simulink model "VehRT_211219"  (R2019b)
settings: Solver=ode5  StartTime=0.0  StopTime=Inf  FixedStep=Ts  RelTol=1e-3  EnableMultiTasking=on
InitFcn:
  | VehRT_Init_211219;
  | Ts=0.0005;
values from neighbouring files (symbols this model uses):
  damping_p = 0.113    [VehRT_Init_211219.m]
  Ff_ab_p = 0.41    [VehRT_Init_211219.m]
  Ff_c_p = 0.4    [VehRT_Init_211219.m]
  friction_enable = 1    [VehRT_Init_211219.m]
  sigma0_p = 200    [VehRT_Init_211219.m]
  sigma1_p = (200)^0.5    (= 14.1421356237)    [VehRT_Init_211219.m]
  td = 0.01    [VehRT_Init_211219.m]
  theta_sb_p = 0.03    [VehRT_Init_211219.m]
undefined symbols (not defined in the file or in its folder): C, canChannel, D, DiscIntNeverNeededParam, g, IO306, Kf, Kr, Lf, Lr, M, magnitude, sigma, trajectory_x11_, trajectory_x12_, trajectory_x13_, trajectory_x14_, trajectory_x15_, trajectory_x16_, trajectory_x17_, trajectory_x21_, trajectory_x22_, trajectory_x23_, trajectory_x24_, trajectory_x25_, trajectory_x26_, trajectory_x27_, trajectory_y11_, trajectory_y12_, trajectory_y13_, trajectory_y14_, trajectory_y15_, trajectory_y16_, trajectory_y17_, trajectory_y21_, trajectory_y22_, trajectory_y23_, trajectory_y24_, trajectory_y25_, trajectory_y26_, trajectory_y27_, zeta
libraries: canmsglib x31, speedgoatlib_IO612 x20, slrtlib x15, simulink x5, speedgoatlib_IO133 x3, xpcutilitieslib x2, canlib x2, xpcrtudplib x2, speedgoatlib_fpga x1, speedgoatlib_fpga_dio x1, autolibshared x1, speedgoatlib_fpga_quadrature x1
(part 3 of 4)

== system VehRT_211219/CEC Vehicle Dynamics 2021/CEC Vehicle Model 2021/ACC_controller ==
  note: V0.0.1 211028 xiataokai 简单PID-ACC速度控制器，0~1加速，-1~0制动
  des_spdKmph : Inport
  acc_mode : Inport  Port=2
  thr_m : Inport  Port=3
  brk_m : Inport  Port=4
  real_spdKmph : Inport  Port=5
  ACC_PID : simulink/Continuous/PID Controller  Controller=PID  Form=Parallel  TimeDomain=Discrete-time  SampleTime=-1  IntegratorMethod=Forward Euler  FilterMethod=Forward Euler  ControllerParametersSource=internal  P=0.11  I=0  D=0.04  UseFilter=on  N=100  TunerSelectOption=Transfer Function Based (PID Tuner App)  InitialConditionSource=internal  InitialConditionForIntegrator=0  InitialConditionForFilter=0  DifferentiatorICPrevScaledInput=0  ExternalReset=none  TrackingMode=off  Kt=1  LimitOutput=on  UpperSaturationLimit=1  LowerSaturationLimit=-2  LinearizeAsGain=on  AntiWindupMode=none  Kb=1  POutMin=[]  POutMax=[]  IOutMin=[]  IOutMax=[]  DOutMin=[]  DOutMax=[]  NOutMin=[]  NOutMax=[]  SumOutMin=[]  SumOutMax=[]  SaturationOutMin=[]  SaturationOutMax=[]  PParamMin=[]  PParamMax=[]  IParamMin=[]  IParamMax=[]  DParamMin=[]  DParamMax=[]  NParamMin=[]  NParamMax=[]  KbParamMin=[]  KbParamMax=[]  KtParamMin=[]  KtParamMax=[]  KbOutMin=[]  KbOutMax=[]  KtOutMin=[]  KtOutMax=[]  IntegratorOutMin=[]  IntegratorOutMax=[]  FilterOutMin=[]  FilterOutMax=[]  SumI1OutMin=[]  SumI1OutMax=[]  SumI2OutMin=[]  SumI2OutMax=[]  SumI3OutMin=[]  SumI3OutMax=[]  SumI4OutMin=[]  SumI4OutMax=[]  SumDOutMin=[]  SumDOutMax=[]  DifferentiatorOutMin=[]  DifferentiatorOutMax=[]  FilterDiffOutCoefMin=[]  FilterDiffOutCoefMax=[]  ReciprocalOutMin=[]  ReciprocalOutMax=[]  SumDenOutMin=[]  SumDenOutMax=[]  SumNumOutMin=[]  SumNumOutMax=[]  DivideOutMin=[]  DivideOutMax=[]  IntegratorContinuousStateAttributes=''  IntegratorStateMustResolveToSignalObject=off  IntegratorRTWStateStorageClass=Auto  FilterContinuousStateAttributes=''  FilterStateMustResolveToSignalObject=off  FilterRTWStateStorageClass=Auto  ParallelPVariant=InternalParameters  IdealPVariant=Disabled  IVariant=InternalParameters  DVariant=InternalParameters  IntegratorVariant=Discrete  SatVariant=Enabled  AWVariant=Passthrough  PCopyVariant=Disabled  TRVariant=Disabled  FdbkBlocksVariant=Forward  IdealPFdbkVariant=Disabled  SatFdbkVariant=Disabled  DerivativeFilterVariant=ForwardEulerFilter  NVariant=InternalParameters  NCopyVariant=Disabled  FilterICVariant=InternalICsFilter  IntegratorICVariant=InternalICs  ExternalResetVariant=Disabled  TRSumVariant=Passthrough  SumFdbkVariant=Disabled  SumVariant=Sum_PID
  Add : Sum  Inputs=+-
  Constant : Constant  Value=0
  Constant1 : Constant  Value=0
  Constant2 : Constant  Value=0
  Gain_brk : Gain  Gain=-1
  Gain_thr : Gain
  LPF : TransferFcn  Denominator=[1/2/pi/1.5 1]
  LT_brk : Lookup_n-D  NumberOfTableDimensions=1  BreakpointsForDimension1=[0, 0.3, 1]  Table=[0, 0.1, 1]  InternalRulePriority=Speed  RndMeth=Simplest  InputSameDT=on
  Switch : Switch  Criteria=u2 > Threshold
  Switch1 : Switch  Criteria=u2 > Threshold
  Switch2 : Switch  Criteria=u2 > Threshold
  Switch_brk : Switch  Criteria=u2 > Threshold
  Switch_thr : Switch  Criteria=u2 > Threshold
  max1_1 : Saturate  UpperLimit=1  LowerLimit=0
  max1_2 : Saturate  UpperLimit=1  LowerLimit=0
  open_loop_comp : Gain  Gain=1.02
  thr : Outport
  brk : Outport  Port=2
  wires:
  des_spdKmph/1 -> open_loop_comp/1
  real_spdKmph/1 -> Add/2
  Add/1 -> Switch/1
  ACC_PID/1 -> LPF/1
  Constant/1 -> Switch_brk/1
  Constant1/1 -> Switch_thr/3
  Switch_brk/1 -> Gain_brk/1
  Gain_brk/1 -> LT_brk/1
  Switch_thr/1 -> Gain_thr/1
  max1_1/1 -> Switch1/1
  Gain_thr/1 -> max1_2/1
  max1_2/1 -> Switch2/1
  LT_brk/1 -> max1_1/1
  LPF/1 -> Switch_thr/1, Switch_thr/2, Switch_brk/3, Switch_brk/2
  open_loop_comp/1 -> Add/1
  Switch/1 -> ACC_PID/1
  Constant2/1 -> Switch/3
  acc_mode/1 -> Switch2/2, Switch1/2, Switch/2
  thr_m/1 -> Switch2/3
  Switch2/1 -> thr/1
  Switch1/1 -> brk/1
  brk_m/1 -> Switch1/3

== system VehRT_211219/CEC Vehicle Dynamics 2021/CEC Vehicle Model 2021/Allocating_T_b ==
  T_brk : Inport
  Selector : Selector  InputPortWidth=4  IndexOptions=Index vector (dialog)  Indices=[1]  OutputSizes=1
  Selector1 : Selector  InputPortWidth=4  IndexOptions=Index vector (dialog)  Indices=[2]  OutputSizes=1
  Selector2 : Selector  InputPortWidth=4  IndexOptions=Index vector (dialog)  Indices=[3]  OutputSizes=1
  Selector3 : Selector  InputPortWidth=4  IndexOptions=Index vector (dialog)  Indices=[4]  OutputSizes=1
  Vector Concatenate : Concatenate  NumInputs=4
  T_b : Outport
  wires:
  Vector Concatenate/1 -> T_b/1
  Selector2/1 -> Vector Concatenate/3
  Selector3/1 -> Vector Concatenate/4
  Selector/1 -> Vector Concatenate/1
  Selector1/1 -> Vector Concatenate/2
  T_brk/1 -> Selector3/1, Selector2/1, Selector/1, Selector1/1

== system VehRT_211219/CEC Vehicle Dynamics 2021/CEC Vehicle Model 2021/Allocating_T_d ==
  T_drv : Inport
  Constant : Constant  Value=0
  Constant1 : Constant  Value=0
  Selector : Selector  InputPortWidth=2  IndexOptions=Index vector (dialog)  Indices=[1]  OutputSizes=1
  Selector1 : Selector  InputPortWidth=2  IndexOptions=Index vector (dialog)  Indices=[2]  OutputSizes=1
  Vector Concatenate : Concatenate  NumInputs=4
  T_d : Outport
  wires:
  Vector Concatenate/1 -> T_d/1
  T_drv/1 -> Selector1/1, Selector/1
  Selector/1 -> Vector Concatenate/1
  Selector1/1 -> Vector Concatenate/2
  Constant/1 -> Vector Concatenate/3
  Constant1/1 -> Vector Concatenate/4

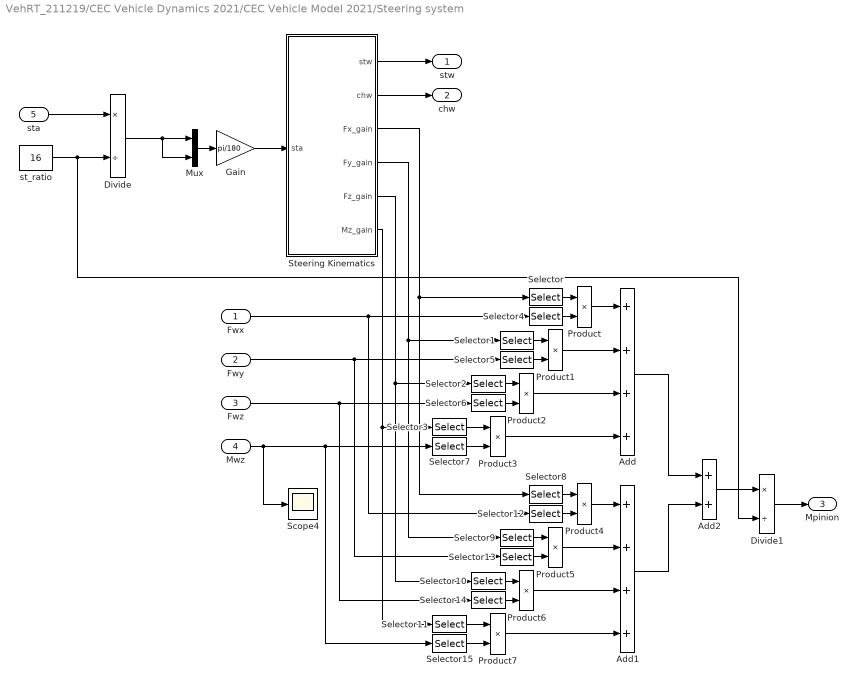
== system VehRT_211219/CEC Vehicle Dynamics 2021/CEC Vehicle Model 2021/Steering system ==
  Fwx : Inport
  Fwy : Inport  Port=2
  Fwz : Inport  Port=3
  Mwz : Inport  Port=4
  sta : Inport  Port=5
  Add : Sum  Inputs=++++
  Add1 : Sum  Inputs=++++
  Add2 : Sum
  Divide : Product  Inputs=*/
  Divide1 : Product  Inputs=*/
  Gain : Gain  Gain=pi/180
  Mux : Mux  Inputs=2
  Product{,1..7} (8 alike) : Product
  Scope4 : Scope
  Selector{,1..3} (4 alike) : Selector  InputPortWidth=2  IndexOptions=Index vector (dialog)  Indices=[1]  OutputSizes=1
  Selector{8..11} (4 alike) : Selector  InputPortWidth=2  IndexOptions=Index vector (dialog)  Indices=[2]  OutputSizes=1
  Selector{12..15} (4 alike) : Selector  InputPortWidth=4  IndexOptions=Index vector (dialog)  Indices=[2]  OutputSizes=1
  Selector{4..7} (4 alike) : Selector  InputPortWidth=4  IndexOptions=Index vector (dialog)  Indices=[1]  OutputSizes=1
  Steering Kinematics : MATLAB Function
  st_ratio : Constant  Value=16
  stw : Outport
  chw : Outport  Port=2
  Mpinion : Outport  Port=3
  wires:
  Gain/1 -> Steering Kinematics/1(sta)
  Mux/1 -> Gain/1
  Divide/1 -> Mux/2, Mux/1
  sta/1 -> Divide/1
  st_ratio/1 -> Divide1/2, Divide/2
  Steering Kinematics/1(stw) -> stw/1
  Steering Kinematics/2(chw) -> chw/1
  Fwx/1 -> Selector12/1, Selector4/1
  Steering Kinematics/3(Fx_gain) -> Selector8/1, Selector/1
  Steering Kinematics/5(Fz_gain) -> Selector10/1, Selector2/1
  Fwz/1 -> Selector14/1, Selector6/1
  Steering Kinematics/6(Mz_gain) -> Selector11/1, Selector3/1
  Mwz/1 -> Scope4/1, Selector15/1, Selector7/1
  Product3/1 -> Add/4
  Product/1 -> Add/1
  Product1/1 -> Add/2
  Product2/1 -> Add/3
  Add/1 -> Add2/1
  Selector/1 -> Product/1
  Selector1/1 -> Product1/1
  Selector2/1 -> Product2/1
  Selector3/1 -> Product3/1
  Selector4/1 -> Product/2
  Selector5/1 -> Product1/2
  Selector6/1 -> Product2/2
  Selector7/1 -> Product3/2
  Add1/1 -> Add2/2
  Selector11/1 -> Product7/1
  Selector12/1 -> Product4/2
  Product6/1 -> Add1/3
  Selector13/1 -> Product5/2
  Selector15/1 -> Product7/2
  Selector9/1 -> Product5/1
  Selector8/1 -> Product4/1
  Selector14/1 -> Product6/2
  Selector10/1 -> Product6/1
  Product7/1 -> Add1/4
  Product4/1 -> Add1/1
  Product5/1 -> Add1/2
  Add2/1 -> Divide1/1
  Steering Kinematics/4(Fy_gain) -> Selector9/1, Selector1/1
  Fwy/1 -> Selector13/1, Selector5/1
  Divide1/1 -> Mpinion/1

== system VehRT_211219/CEC Vehicle Dynamics 2021/CEC Vehicle Model 2021/Vehicle_initializer ==
  spd0Kmph : Inport
  MATLAB Function : MATLAB Function  TreatAsAtomicUnit=on
  pwrXInit : Outport
  gearInit : Outport  Port=2
  tirInit : Outport  Port=3
  vehInit : Outport  Port=4
  wires:
  spd0Kmph/1 -> MATLAB Function/1(V)
  MATLAB Function/1(gearInit) -> gearInit/1
  MATLAB Function/3(pwrXInit) -> pwrXInit/1
  MATLAB Function/4(tirXInit) -> tirInit/1
  MATLAB Function/2(vehXInit) -> vehInit/1

== system VehRT_211219/CEC Vehicle Dynamics 2021/CEC Vehicle Model 2021/awCal ==
  In1 : Inport
  Selector_aw : Selector  InputPortWidth=8  IndexOptions=Index vector (dialog)  Indices=[5:8]  OutputSizes=1
  atan_and_r2d : MATLAB Function  TreatAsAtomicUnit=on
  y : Outport
  wires:
  In1/1 -> Selector_aw/1
  Selector_aw/1 -> atan_and_r2d/1(u)
  atan_and_r2d/1(y) -> y/1

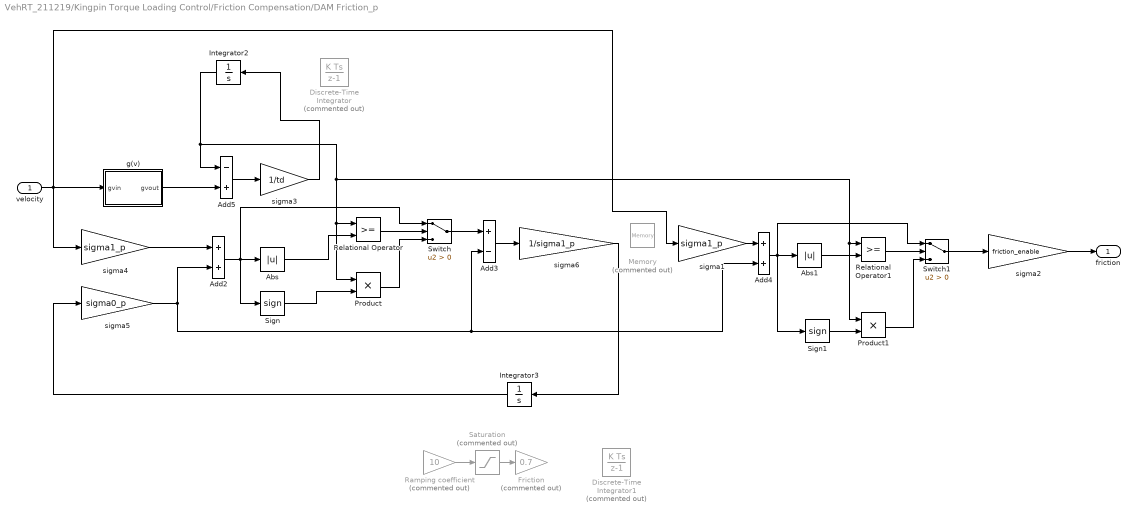
== system VehRT_211219/Kingpin Torque Loading Control/Friction Compensation/DAM Friction_p ==
  velocity : Inport
  Abs : Abs
  Abs1 : Abs
  Add2 : Sum
  Add3 : Sum  Inputs=+-
  Add4 : Sum
  Add5 : Sum  Inputs=-+
  Discrete-Time Integrator : DiscreteIntegrator  Commented=on  SampleTime=-1  ICPrevOutput=DiscIntNeverNeededParam  ICPrevScaledInput=DiscIntNeverNeededParam
  Discrete-Time Integrator1 : DiscreteIntegrator  Commented=on  SampleTime=-1  LimitOutput=on  UpperSaturationLimit=Ff_ab_p/sigma0_p  LowerSaturationLimit=-Ff_ab_p/sigma0_p  ICPrevOutput=DiscIntNeverNeededParam  ICPrevScaledInput=DiscIntNeverNeededParam
  Friction : Gain  Commented=on  Gain=0.7
  Integrator2 : Integrator
  Integrator3 : Integrator  LimitOutput=on  UpperSaturationLimit=Ff_ab_p/sigma0_p  LowerSaturationLimit=-Ff_ab_p/sigma0_p
  Memory : Memory  Commented=on
  Product : Product  RndMeth=Zero
  Product1 : Product  RndMeth=Zero
  Ramping coefficient : Gain  Commented=on  Gain=10
  Relational Operator : RelationalOperator  OutDataTypeStr=boolean  RndMeth=Nearest
  Relational Operator1 : RelationalOperator  OutDataTypeStr=boolean  RndMeth=Nearest
  Saturation : Saturate  Commented=on  UpperLimit=1  LowerLimit=-1
  Sign : Signum
  Sign1 : Signum
  Switch : Switch  Criteria=u2 > Threshold
  Switch1 : Switch  Criteria=u2 > Threshold
  g(v) : Subsystem
  sigma1 : Gain  Gain=sigma1_p
  sigma2 : Gain  Gain=friction_enable
  sigma3 : Gain  Gain=1/td
  sigma4 : Gain  Gain=sigma1_p
  sigma5 : Gain  Gain=sigma0_p
  sigma6 : Gain  Gain=1/sigma1_p
  friction : Outport  VectorParamsAs1DForOutWhenUnconnected=off
  wires:
  Relational Operator1/1 -> Switch1/2
  Abs1/1 -> Relational Operator1/2
  sigma1/1 -> Add4/1
  Integrator3/1 -> sigma5/1
  Add3/1 -> sigma6/1
  Switch/1 -> Add3/1
  Product/1 -> Switch/3
  Sign/1 -> Product/2
  Relational Operator/1 -> Switch/2
  Abs/1 -> Relational Operator/2
  Add2/1 -> Sign/1, Switch/1, Abs/1
  sigma6/1 -> Integrator3/1
  sigma5/1 -> Add2/2, Add3/2, Add4/2
  sigma4/1 -> Add2/1
  Add5/1 -> sigma3/1
  g(v)/1(gvout) -> Add5/2
  Switch1/1 -> sigma2/1
  sigma2/1 -> friction/1
  sigma3/1 -> Integrator2/1
  velocity/1 -> sigma1/1, sigma4/1, g(v)/1(gvin)
  Product1/1 -> Switch1/3
  Sign1/1 -> Product1/2
  Add4/1 -> Sign1/1, Switch1/1, Abs1/1
  Integrator2/1 -> Product1/1, Relational Operator1/1, Product/1, Relational Operator/1, Add5/1
  Saturation/1 -> Friction/1
  Ramping coefficient/1 -> Saturation/1

== system VehRT_211219/Kingpin Torque Loading Control/Old baks/Aligning Torque Calculator ==
  Beta : Inport
  r : Inport  Port=2
  Fzf : Inport  Port=3
  speed : Inport  Port=4
  Delta : Inport  Port=5
  Add3 : Sum  Inputs=++-
  Add4 : Sum
  Divide1 : Product  Inputs=*/
  Divide2 : Product  Inputs=**
  Gain : Gain  Gain=2
  Gain1 : Gain  Gain=Lf
  Gain2 : Gain  Gain=2*zeta*Kf
  Gain5 : Gain  Gain=0.5*D*sin(2*sigma)
  Trigonometric Function : Trigonometry
  Tire Aligning Torque : Outport  VectorParamsAs1DForOutWhenUnconnected=off
  wires:
  r/1 -> Gain1/1
  Gain1/1 -> Divide1/1
  speed/1 -> Divide1/2
  Delta/1 -> Trigonometric Function/1, Add3/3  "Delta"
  Beta/1 -> Add3/2
  Divide1/1 -> Add3/1
  Add3/1 -> Gain2/1
  Trigonometric Function/1 -> Divide2/1
  Divide2/1 -> Gain5/1
  Gain2/1 -> Add4/1
  Gain5/1 -> Add4/2
  Add4/1 -> Tire Aligning Torque/1
  Gain/1 -> Divide2/2
  Fzf/1 -> Gain/1

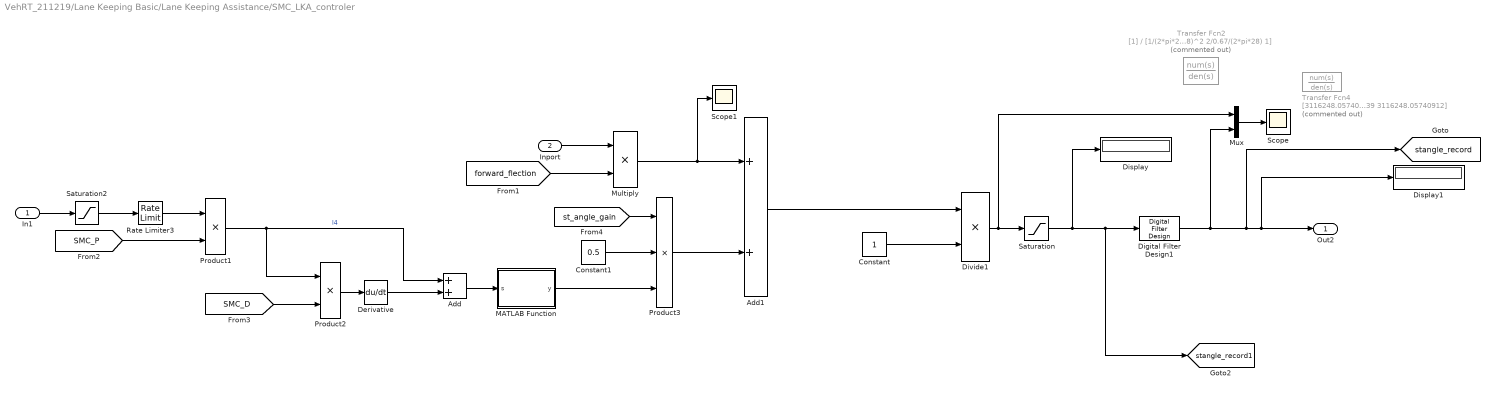
== system VehRT_211219/Lane Keeping Basic/Lane Keeping Assistance/SMC_LKA_controler ==
  In1 : Inport
  Inport : Inport  Port=2
  Add : Sum
  Add1 : Sum
  Constant : Constant
  Constant1 : Constant  Value=0.5
  Derivative : Derivative
  Digital Filter Design1 : dsparch4/Digital Filter Design  mwdsp_browser_bugfix_var=off
  Display : Display
  Display1 : Display
  Divide1 : Product  Inputs=**
  MATLAB Function : MATLAB Function  TreatAsAtomicUnit=on
  Multiply : Product
  Mux : Mux  Inputs=2
  Product1 : Product
  Product2 : Product
  Product3 : Product  Inputs=3
  Rate Limiter3 : RateLimiter  RisingSlewLimit=25  FallingSlewLimit=-25  SampleTimeMode=inherited
  Saturation : Saturate  UpperLimit=60  LowerLimit=-60
  Saturation2 : Saturate  UpperLimit=4  LowerLimit=-4
  Scope : Scope
  Scope1 : Scope
  Transfer Fcn2 : TransferFcn  Commented=on  Denominator=[1/(2*pi*28)^2 2/0.67/(2*pi*28) 1]
  Transfer Fcn4 : TransferFcn  Commented=on  Numerator=[3116248.05740912]  Denominator=[1 292.128549685798 42669.5447707639 3116248.05740912]
  Out2 : Outport  VectorParamsAs1DForOutWhenUnconnected=off
  tag scope: stangle_record1=global, stangle_record=global
  wires:
  Product3/1 -> Add1/2
  Add/1 -> MATLAB Function/1(s)
  Derivative/1 -> Add/2
  Product1/1 -> Add/1, Product2/1  "l4"
  Product2/1 -> Derivative/1
  [SMC_D] -> Product2/2
  Constant1/1 -> Product3/2
  [st_angle_gain] -> Product3/1
  MATLAB Function/1(y) -> Product3/3
  Add1/1 -> Divide1/1
  Divide1/1 -> Saturation/1, Mux/1
  Mux/1 -> Scope/1
  Constant/1 -> Divide1/2
  Multiply/1 -> Scope1/1, Add1/1
  Inport/1 -> Multiply/1
  [SMC_P] -> Product1/2
  Saturation2/1 -> Rate Limiter3/1
  In1/1 -> Saturation2/1
  [forward_flection] -> Multiply/2
  Rate Limiter3/1 -> Product1/1
  Digital Filter Design1/1 -> [stangle_record], Display1/1, Out2/1, Mux/2
  Saturation/1 -> Digital Filter Design1/1, [stangle_record1], Display/1

== system VehRT_211219/Lane Keeping Basic/Lane Keeping Assistance/signal processing ==
  Demux : Demux  Outputs=2
  Display : Display
  Gain : Gain
  Mux : Mux  Inputs=2
  Mux1 : Mux  Inputs=2
  Relational Operator : RelationalOperator  Operator=>  OutDataTypeStr=boolean  RndMeth=Simplest
  Saturation : Saturate  UpperLimit=4  LowerLimit=-4
  Switch : Switch  Criteria=u2 > Threshold  Threshold=0.5
  loading scope : slrtlib/Displays and Logging/Scope   scopeno=2  scopetype=Target  autostart=on  viewmode=Graphical rolling  formatstr='%15.6f'  grid=on  ylimits=[-5,5]  nosamples=1000  noprepostsamples=0  interleave=1  triggermode=FreeRun  triggersignal=1  trigsignalfromport=off  triggerlevel=0.0  triggerslope=Either  triggerscope=1  triggersample=0  filename=data.dat  mode=Lazy  writesize=512  autorestart=off  dynamicfilemode=off  maxwritefilesize=512*1024^2
  path_following : MATLAB Function  TreatAsAtomicUnit=on
  prepoint_y : Subsystem
  offset_at_prviewtime1 : Outport  VectorParamsAs1DForOutWhenUnconnected=off
  qulv_at_prviewtime2 : Outport  Port=2  VectorParamsAs1DForOutWhenUnconnected=off
  tag scope: offset_record=global, select_flag=global
  wires:
  prepoint_y/2(Out2) -> Relational Operator/1, path_following/4(prey)
  [trajectory_x] -> path_following/1(u)
  [trajectory_y] -> path_following/2(w)
  path_following/1(Y) -> Mux/1
  path_following/2(qulv) -> Mux/2
  prepoint_y/1(Out1) -> path_following/3(prex)
  [deviation_from_prescan] -> Saturation/1, Display/1
  [qulv_from_prescan] -> Mux1/2
  Demux/1 -> [offset_record], offset_at_prviewtime1/1
  Demux/2 -> qulv_at_prviewtime2/1
  [theend] -> Relational Operator/2
  Mux/1 -> Switch/1
  Mux1/1 -> Switch/3
  Relational Operator/1 -> [select_flag], Switch/2
  Gain/1 -> Mux1/1
  Switch/1 -> Demux/1
  Saturation/1 -> loading scope/1, Gain/1

== system VehRT_211219/Lane Keeping Basic/SMC characters/Subsystem ==
  Constant1 : Constant  Value=3.5
  Constant10 : Constant  Value=2.15
  Constant11 : Constant  Value=0.008
  Constant15 : Constant  Value=2000
  Constant2 : Constant  Value=0.01
  Constant3 : Constant  Value=930
  Constant4 : Constant  Value=5.5
  Constant9 : Constant  Value=8
  Memory : Memory
  Mux : Mux  Inputs=5
  Mux1 : Mux  Inputs=5
  Switch : Switch  Criteria=u2 > Threshold  Threshold=0.5
  st_angle_max : Constant  Value=40
  st_angle_max1 : Constant  Value=180
  Out1 : Outport  VectorParamsAs1DForOutWhenUnconnected=off
  wires:
  Mux/1 -> Switch/3
  Constant9/1 -> Mux/2
  Constant10/1 -> Mux/3
  Constant11/1 -> Mux/4
  st_angle_max/1 -> Mux/5
  Constant15/1 -> Mux/1
  Switch/1 -> Out1/1
  Constant3/1 -> Mux1/1
  st_angle_max1/1 -> Mux1/5
  Constant2/1 -> Mux1/4
  Constant1/1 -> Mux1/3
  Constant4/1 -> Mux1/2
  Mux1/1 -> Switch/1
  Memory/1 -> Switch/2
  [select_flag] -> Memory/1

== system VehRT_211219/Lane Keeping Basic/SMC characters/Subsystem2 ==
  Constant1 : Constant  Value=250
  Constant10 : Constant  Value=1.5
  Constant11 : Constant  Value=0.12
  Constant9 : Constant  Value=24
  Mux : Mux  Inputs=5
  st_angle_max : Constant  Value=30
  Out1 : Outport  VectorParamsAs1DForOutWhenUnconnected=off
  wires:
  Mux/1 -> Out1/1
  st_angle_max/1 -> Mux/5
  Constant11/1 -> Mux/4
  Constant9/1 -> Mux/2
  Constant10/1 -> Mux/3
  Constant1/1 -> Mux/1

== system VehRT_211219/Kingpin Torque Loading Control/Friction Compensation/DAM Friction_p/g(v) ==
  gvin : Inport
  Add4 : Sum  Inputs=-+
  Add5 : Sum
  Constant1 : Constant  Value=Ff_c_p
  Constant4 : Constant  Value=theta_sb_p
  Constant5 : Constant  Value=2
  Constant6 : Constant  Value=Ff_ab_p
  Divide1 : Product  Inputs=*/
  Math Function : Math  SaturateOnIntegerOverflow=on
  Math Function1 : Math  Operator=pow  SaturateOnIntegerOverflow=on
  Product1 : Product  RndMeth=Zero
  Scope3 : Scope
  sigma3 : Gain  Gain=-1
  gvout : Outport  VectorParamsAs1DForOutWhenUnconnected=off
  wires:
  Add5/1 -> gvout/1
  Constant4/1 -> Divide1/2
  Divide1/1 -> Math Function1/1
  Constant5/1 -> Math Function1/2
  sigma3/1 -> Math Function/1
  Math Function1/1 -> sigma3/1
  Math Function/1 -> Product1/1
  Constant6/1 -> Add4/2
  Add4/1 -> Product1/2
  Product1/1 -> Scope3/1, Add5/1
  Constant1/1 -> Add4/1, Add5/2
  gvin/1 -> Divide1/1

== system VehRT_211219/Lane Keeping Basic/Lane Keeping Assistance/signal processing/prepoint_y ==
  Fcn : Fcn  Expr=u-1056
  Fcn1 : Fcn  Expr=-u+78.486
  Fcn2 : Fcn  Expr=-u
  MATLAB Function1 : MATLAB Function  TreatAsAtomicUnit=on
  Out1 : Outport  VectorParamsAs1DForOutWhenUnconnected=off
  Out2 : Outport  Port=2  VectorParamsAs1DForOutWhenUnconnected=off
  wires:
  [Yaw] -> Fcn2/1
  [X] -> Fcn/1
  [Y] -> Fcn1/1
  [road_id_from_precan] -> MATLAB Function1/4(road_id)
  MATLAB Function1/1(xp) -> Out1/1
  MATLAB Function1/2(yp) -> Out2/1
  [prepoint_distance] -> MATLAB Function1/5(preview_dis)
  Fcn2/1 -> MATLAB Function1/3(local_yaw)
  Fcn/1 -> MATLAB Function1/1(local_x)
  Fcn1/1 -> MATLAB Function1/2(local_y)

== matlab function VehRT_211219/Hardware Interfaces/Torque Switch Interface /torque switch ==
  data: button_on input; control output; button_off input
function control = digiin(button_on,button_off)
persistent on_old
persistent off_old
persistent state
if isempty(on_old)
    on_old = 1;
    off_old = 1;
    state = 0;
end
if state == 0 &&(on_old > 0.5 && button_on < 0.5)
    state = 1;
elseif state == 1 &&(off_old > 0.5 && button_off < 0.5)
    state = 0;
end
control = state;

== matlab function VehRT_211219/Kingpin Torque Loading Control/Postion Process (double datatype) ==
  data: pos_input input; pos_output output; spd_output output; t input
function [pos_output,spd_output] = fcn(pos_input,t)
persistent pos_old
persistent spd_old
persistent t_old
persistent SPR
if isempty(pos_old) || t<0.3
    SPR = double(6815744/2);
    t_old = t;
    pos_old = double(0);
    spd_old = double(0);
    pos_output = 0;
    spd_output = 0;
else
    pos_input = double(pos_input);
    dt = t-t_old;
    error = pos_input-pos_old;
    % huge step between two neighbor signals in one time series is not allowed
    edge_crossing = floor((abs(error)+SPR/2)./SPR).*(-sign(error)); 
    pos_new = edge_crossing*SPR + pos_input;
    pos_output = double(pos_new)/double(SPR)*360;  % unit: deg
    spd_output = double(pos_new-pos_old)/double(SPR)*360/dt; % unit: deg per second
    if abs(spd_output-spd_old)>700 % speed calculation glitch prevetion
        spd_output = spd_old;
    end
    t_old = t;
    pos_old = pos_new;
    spd_old = spd_output;
end

== matlab function VehRT_211219/EPS Steering Torque Assist Control/Assist Curve ==
  data: turn input; relative_center_gain input; in input; out output; V input
function out = fcn(turn,relative_center_gain,in,V)
main_gain = min(max(-0.018*V+1.8,0),1);
if abs(in)>abs(turn)
    out = in+sign(in)*(turn*(relative_center_gain-1));
else
    out = relative_center_gain*in;
end
out = main_gain*out;

== matlab function VehRT_211219/Connect Scenery/MATLAB Function ==
  data: origin input; interval output; feedback input; delay output
function [interval,delay] = analysis(origin,feedback)
persistent origin_buffer
persistent feedback_buffer
persistent flag1
persistent flag2
% 超参数
buffer_length = 10000;
step_time = 1;
tolerance = 25;
% 变量初始化
if isempty(origin_buffer)
    origin_buffer = zeros(1,buffer_length);
    feedback_buffer = zeros(1,buffer_length);
    flag1 = int32(0);
    flag2 = 0;
end
%存入新的数据
flag1 = flag1+1;
if flag1>buffer_length
    flag1 = int32(1);
    flag2 = 1;
end
origin_buffer(flag1)=origin;
feedback_buffer(flag1)=feedback;
%向前搜索相同的点，直至buffer有效范围尽头
flag3 = 0;
flag4 = 0;
feedback_index = flag1+1;
origin_index = flag1+1;
if flag2 == 0
    range = flag1:-1:1;
else
    range = [flag1:-1:1,buffer_length:-1:(flag1+1)];
end
breakflag = 0;
for tag = 1:length(range)
    if flag3 == 0 && feedback~=feedback_buffer(range(tag))
        flag3 = 1;
        feedback_index = range(tag);
        breakflag = breakflag+1;
    end
    if flag4 == 0 && abs(feedback-origin_buffer(range(tag)))<tolerance
        flag4 = 1;
        origin_index = range(tag);
        breakflag = breakflag+1;
    end
    if breakflag>1
        break;
    end
end
%计算延时与数据帧间隔
interval = double(buffer_length)*step_time;
if flag3 ~=0
    if feedback_index<=flag1
        interval = double((flag1-feedback_index+1))*step_time;
    else
        interval = double(((flag1-1)+(buffer_length+1-feedback_index)+1))*step_time;
    end
end
delay = double(buffer_length)*step_time;
if flag4 ~=0
    if origin_index<=flag1
        delay = double((flag1-origin_index+1))*step_time;
    else
        delay = double(((flag1-1)+(buffer_length+1-origin_index)+1))*step_time;
    end
end
end

== matlab function VehRT_211219/EPS Steering Torque Assist Control/Damping Control Strategy ==
  settings: updateMethod=DISCRETE
  data: spd input; control output; ang input
function control = fcn(spd,ang)
persistent state
persistent spd_old
if isempty(state)
    state = 0;
    spd_old =spd;
end
if state==0
    if -sign(ang)*sign(spd)>0 && abs(ang)>20
        state =1;
    end
else
    if sign(spd_old)*sign(spd)>0
        state = 1;
    else
        state = 0;
    end
end
spd_old = spd;
control = state*abs(spd);

== matlab function VehRT_211219/Hardware Interfaces/Postion Process (double datatype) ==
  data: pos_input input; pos_output output
function pos_output  = fcn(pos_input)
persistent pos_old
persistent SPR
if isempty(pos_old)
    SPR = double(360);
    pos_old = double(0);
    pos_output = 0;
else
    pos_input = double(pos_input);
    error = pos_input-pos_old;
    % huge step between two neighbor signals in one time series is not allowed
    edge_crossing = floor((abs(error)+SPR/2)./SPR).*(-sign(error)); 
    pos_new = edge_crossing*SPR + pos_input;
    pos_output = double(pos_new)/double(SPR)*360;  % unit: deg
    pos_old = pos_new;
end

== matlab function VehRT_211219/CEC Vehicle Dynamics 2021/CEC Vehicle Model 2021/Brake ==
  settings: updateMethod=DISCRETE
  data: X input; X_dot output; per input; u input; kw input; T_brk output
% 制动系统模型（液压制动、简单ABS）
% V0.0.2 20211015 xiataokai ABS基本功能

function [X_dot, T_brk] = brk(X, per, u, kw)
% u is in km/h
% Pedal percentage to pedal force, (-, N)
f_pedal = [0, 0; 1, 900];
% Pedal force to booster force, (N, N)
f_boost = [0, 0; 70, 0; 75, 75; 700, 3550; 900, 3750];
% Pedal lever ratio, -
r_lever = 4.1;
% M/C diameter, mm
D = 25;
% Time constants for booster dynamics, s
T_app = 0.16;
T_rel = 0.07;
% ABS type for front and rear axle
ch_F = 2;
ch_R = 1;
% ABS parameters for front axle, longitudinal slip for turning the brake, -
abs_slip_off_F = 0.1;
abs_slip_on_F = 0.05;
% ABS parameters for front axle, minimum vehicle speed, km/h
abs_vmin_F = 3;
% ABS parameters for rear axle, longitudinal slip for turning the brake, -
abs_slip_off_R = 0.1;
abs_slip_on_R = 0.05;
% ABS parameters for rear axle, minimum vehicle speed, km/h
abs_vmin_R = 3;
% Delivery/line pressure ratio for front axle, -
pbk_dl_F = 1;
% Delivery/line pressure ratio for rear axle, -
pbk_dl_R = 0.4;
% Actuator time constant for front axle, s
T_bk_F = 0.06;
% Actuator time constant for rear axle, s
T_bk_R = 0.06;
% Torque/pressure coefficient for front axle, N-m/MPa
tbk_pbk_F = 150;
% Torque/pressure coefficient for rear axle, N-m/MPa
tbk_pbk_R = 100;
% Bearing/brake friction for front axle, N-m
tbk_c_F = 0.5;
% Bearing/brake friction for rear axle, N-m
tbk_c_R = 0.5;


% Persistent brake states
persistent abs_b;
persistent per_old;
if isempty(abs_b)
    abs_b = ones(4,1);
    per_old = per;
end

% ABS controller logic
if u < abs_vmin_F
    abs_b(1) = 1;
    abs_b(2) = 1;
else
    if ch_F == 1
       if(abs_b(1) == 1 && (abs(kw(1)) > abs_slip_off_F || abs(kw(2)) > abs_slip_off_F)) 
           abs_b(1) = 0;
           abs_b(2) = 0;
       elseif(abs_b(1) == 0 && abs(kw(1)) < abs_slip_on_F && abs(kw(2)) < abs_slip_on_F)
           abs_b(1) = 1;
           abs_b(2) = 1;
       end
    else
       if(abs_b(1) == 1 && abs(kw(1)) > abs_slip_off_F) 
           abs_b(1) = 0;
       elseif(abs_b(1) == 0 && abs(kw(1)) < abs_slip_on_F)
           abs_b(1) = 1;
       end
       if(abs_b(2) == 1 && abs(kw(2)) > abs_slip_off_F) 
           abs_b(2) = 0;
       elseif(abs_b(2) == 0 && abs(kw(2)) < abs_slip_on_F)
           abs_b(2) = 1;
       end
    end
end
if u < abs_vmin_R
    abs_b(3) = 1;
    abs_b(4) = 1;
else
    if ch_R == 1
       if(abs_b(3) == 1 && (abs(kw(3)) > abs_slip_off_R || abs(kw(4)) > abs_slip_off_R)) 
           abs_b(3) = 0;
           abs_b(4) = 0;
       elseif(abs_b(3) == 0 && abs(kw(3)) < abs_slip_on_R && abs(kw(4)) < abs_slip_on_R)
           abs_b(3) = 1;
           abs_b(4) = 1;
       end
    else
       if(abs_b(3) == 1 && abs(kw(3)) > abs_slip_off_R) 
           abs_b(3) = 0;
       elseif(abs_b(3) == 0 && abs(kw(3)) < abs_slip_on_R)
           abs_b(3) = 1;
       end
       if(abs_b(4) == 1 && abs(kw(4)) > abs_slip_off_R) 
           abs_b(4) = 0;
       elseif(abs_b(4) == 0 && abs(kw(4)) < abs_slip_on_R)
           abs_b(4) = 1;
       end
    end
end

% Cylinder pressure dynamic
F_mc = X(5);
F_pedal = intMap1(f_pedal, per);
if per >= per_old
    F_mc_dot = (intMap1(f_boost, F_pedal*r_lever) - F_mc)/T_app*2*pi;
else
    F_mc_dot = (intMap1(f_boost, F_pedal*r_lever) - F_mc)/T_rel*2*pi;
end
pbk_con = F_mc/pi/D^2*4; % pbk_con is in MPa
X_dot = zeros(5,1);
X_dot(5) = F_mc_dot;

% Delivery pressure proportioning
pbk_LF_ctl = pbk_con * pbk_dl_F * abs_b(1);
pbk_RF_ctl = pbk_con * pbk_dl_F * abs_b(2);
pbk_LR_ctl = pbk_con * pbk_dl_R * abs_b(3);
pbk_RR_ctl = pbk_con * pbk_dl_R * abs_b(4);

% Actuator dynamics
pbk_LF = X(1);
pbk_RF = X(2);
pbk_LR = X(3);
pbk_RR = X(4);
pbk_LF_dot = (pbk_LF_ctl - pbk_LF)/T_bk_F*2*pi;
pbk_RF_dot = (pbk_RF_ctl - pbk_RF)/T_bk_F*2*pi;
pbk_LR_dot = (pbk_LR_ctl - pbk_LR)/T_bk_R*2*pi;
pbk_RR_dot = (pbk_RR_ctl - pbk_RR)/T_bk_R*2*pi;
X_dot(1) = pbk_LF_dot;
X_dot(2) = pbk_RF_dot;
X_dot(3) = pbk_LR_dot;
X_dot(4) = pbk_RR_dot;

% Brake torque at wheels
T_brk = zeros(4,1);
T_brk(1) = pbk_LF * tbk_pbk_F + tbk_c_F;
T_brk(2) = pbk_RF * tbk_pbk_F + tbk_c_F;
T_brk(3) = pbk_LR * tbk_pbk_R + tbk_c_R;
T_brk(4) = pbk_RR * tbk_pbk_R + tbk_c_R;
end

% 1D-Map interp
function v1 = intMap1(V, x0)
if x0 <= V(1,1)
    v1 = V(1,2);
elseif x0 >= V(end,1)
    v1 = V(end,2);
else
    for i = 1:size(V,1)-1
        if V(i+1,1) > x0; break; end
    end
    v1 = V(i,2)*(V(i+1,1)-x0)/(V(i+1,1)-V(i,1))+V(i+1,2)*(x0-V(i,1))/(V(i+1,1)-V(i,1));
end
end

== matlab function VehRT_211219/CEC Vehicle Dynamics 2021/Reset with Clutch/Reset Funvtion ==
  settings: updateMethod=DISCRETE
  data: clt input; t input; rst output
function rst =fcn(clt, t)
persistent clt_old
persistent rst_state
persistent t_old
if isempty(clt_old)
    clt_old =0;
    rst_state = 0;
    t_old = t;
end
if ((clt_old <40 && clt>=40 && rst_state == 0) || (clt>=40 && rst_state == 1))
    t_old = t;
end
if (clt>=40 && rst_state == 0 && (t-t_old)>2.56)
    rst_state = 1;
end
if (clt < 40 && rst_state == 1 && (t-t_old)>0.5)
    rst_state = 0;
end

clt_old = clt;
rst = rst_state;

== matlab function VehRT_211219/CEC Vehicle Dynamics 2021/CEC Vehicle Model 2021/Powertrain ==
  settings: updateMethod=DISCRETE
  data: X input; t input; X_dot output; thr input; wg0 input; Ag0 input; T_drv output; I_drv output; gr output; weng output; wtran output; Stc output; Te output; Ttcin output; Ttcout output; gr_init input
% 动力总成模型（150kW发动机、液力变矩器、6AT变速箱、开放差速器）
% V0.0.2 20211013 xiataokai 换挡逻辑修正，加入传动轴惯量变化考虑

function [X_dot, T_drv, I_drv, gr, weng, wtran, Stc, Te, Ttcin, Ttcout] = pwr(X, t, thr, wg0, Ag0 ,gr_init)
% Engine torque map (N-m. - , rpm) (engine torque . throtle , engine speed)
Eng1 = [0,0,0,0,0,0,0,0,0,0;0,0,0,0,0,0,0,0,0,0;... 
    24.7500,76.1100,101.370,103.430,104.600,105.180,105.380,105.430,105.460,105.430;
    29.7000,92.8700,139.660,149.150,150.670,151.280,151.500,151.520,151.520,151.520;
    0,87.3900,148.020,161.350,164.950,166.250,166.730,166.770,166.770,166.750;
    -9.9000,70.6200,173.590,198.660,208.610,212.020,213.290,213.400,213.370,213.290;
    -14.8500,47.1200,167.310,207.900,221.150,227.150,230.090,230.770,231.220,235.620;
    -16.8300,25.7400,148.500,211.600,233.680,242.290,246.890,248.140,249.060,255.420;
    -20.1700,9.90000,117.650,203.670,237.600,257.400,260.370,263.340,266.310,272.880;
    -25.3200,-6.41000,81.3000,182.080,239.580,267,274.230,279.240,282.150,287.100;
    -30.1400,-15.1600,56.4100,153.500,233.120,269.900,285.220,289.080,295.020,299.970;
    -34.3900,-22.0600,37.6600,122.490,223.450,267.300,287.100,295.020,300.960,306.900;
    -38.5700,-28.1000,23.4800,96.5300,201.040,259.380,288.090,297,303.930,309.870;
    -42.7700,-33.7100,11.8000,76.4200,174.350,248.620,285.120,296.010,302.940,306.900;
    -47.2100,-39.3800,0.280000,57.4500,150.240,237.300,280.170,290.070,297,302.880;
    -51.8300,-45.0100,-9.97000,41.1900,125.060,220.310,272.250,282.150,292.050,297;
    -56.7400,-50.5700,-19.0800,26.9900,102.650,198.960,262.350,272.250,282.150,287.100;
    -61.6700,-56.2400,-27.5300,14.4500,83.5200,176.580,246.840,256.410,269.640,272.490;
    -67.1900,-62.1700,-35.7200,2.82000,66.2000,153.280,221.410,236.520,243.610,246.410;
    -73.2100,-68.4100,-43.8800,-8.16000,50.3800,130.660,193.860,207.920,214.520,217.050;
    -80.1900,-80.1900,-80.1900,-80.1900,-80.1900,-80.1900,-80.1900,-80.1900,-80.1900,-80.1900;
    -81.1800,-81.1800,-81.1800,-81.1800,-81.1800,-81.1800,-81.1800,-81.1800,-81.1800,-81.1800];
% Engine torque map throttle
Eng1_thr = [0,0.10,0.15,0.20,0.35,0.50,0.70,0.85,0.95,1];
% Engine torque map rpm
Eng1_rpm = [0;400;517;633;750;1107;1463;1820;2177;2533;2890;3247;3603;3960;4317;4673;5030;5387;5743;6100;6500;6700];
% Engine crankshaft spin inertia, kg-m2
Eng1_I = 0.2; 

% Torque convertor inverse capacity factor 1/K (- , sqrt[N-m]/rpm) (speed ratio , 1/K)
TC1_tki = [0,0.00704273;0.100000,0.00704273;0.200000,0.00704273;0.300000,0.00704269;
    0.400000,0.00704199;0.500000,0.00703585;0.600000,0.00700014;0.700000,0.00684379;
    0.800000,0.00628652;0.900000,0.00458708;0.950000,0.00282599;0.990000,0.000673411;
    1.01000,-0.000673411;1.05000,-0.00282599;1.10000,-0.00458708;1.20000,-0.00628652;
    1.30000,-0.00684379;1.40000,-0.00700014;1.50000,-0.00703585;1.60000,-0.00704199;
    1.70000,-0.00704269;1.80000,-0.00704273;1.90000,-0.00704273;2,-0.00704273];
% Torque converter torque ratio (- , -) (speed ratio , torque ratio)
TC1_tr = [0,1.86400;0.88100,1;1,1];
% Torque converter input shaft spin inertia, kg-m2
TC1_Iis = 0.015;
% Torque converter output shaft spin inertia, kg-m2
TC1_Ios = 0.015;

% Transmission gear ratio, - (gear1 ~ gear6)
Trans1_N = [3.538, 2.060, 1.404, 1.000, 0.713, 0.582];
% Transmission inertia, kg-m2 (gear1 ~ gear6)
Trans1_I = [0.037, 0.034, 0.042, 0.040, 0.040, 0.040];
% Transmission efficiency when driving, - (gear1 ~ gear6)
Trans1_ed = [0.920, 0.920, 0.950, 0.950, 0.980, 0.990];
% Transmission efficiency when coasting, - (gear1 ~ gear6)
Trans1_ec = [0.920, 0.920, 0.950, 0.950, 0.980, 0.990];
% Transmission shift duration legacy, s
Trans1_legacy = 0.25;
% Transmission shift shedule 1-2 (- , rpm) (throttle , output speed in lower gear)
Trans1_u12 = [0, 874; 0.2, 874; 0.8, 1653; 1, 1653]; 
Trans1_d21 = [0. 699; 0.4, 699; 0.8, 1240; 1, 1240]; 
% Transmission shift shedule 2-3 (- , rpm) (throttle , output speed in lower gear)
Trans1_u23 = [0, 1282; 0.2, 1282; 0.8, 2840; 1, 2840];
Trans1_d32 = [0. 1026; 0.4, 1026; 0.8, 2130; 1, 2130];
% Transmission shift shedule 3-4 (- , rpm) (throttle , output speed in lower gear)
Trans1_u34 = [0, 1800; 0.2, 1800; 0.8, 4167; 1, 4167];
Trans1_d43 = [0. 1440; 0.4, 1440; 0.8, 3125; 1, 3125];
% Transmission shift shedule 4-5 (- , rpm) (throttle , output speed in lower gear)
Trans1_u45 = [0, 2525; 0.2, 2525; 0.8, 5850; 1, 5850];
Trans1_d54 = [0. 2020; 0.4, 2020; 0.8, 4388; 1, 4388];
% Transmission shift shedule 5-6 (- , rpm) (throttle , output speed in lower gear)
Trans1_u56 = [0, 3093; 0.2, 3093; 0.8, 8205; 1, 8205];
Trans1_d65 = [0. 2474; 0.4, 2474; 0.8, 6154; 1, 6154];
% Transmission shedule collection
Trans1_u = {Trans1_u12, Trans1_u23, Trans1_u34, Trans1_u45, Trans1_u56};
Trans1_d = {Trans1_d21, Trans1_d32, Trans1_d43, Trans1_d54, Trans1_d65};

% Differential gear ratio, -
Diff_N = 5.0; % 4.1
% Differential drive shaft inertial, kg-m2
Diff_Ishaft = 0.013;
% Differential shaft to left wheel intertial, kg-m2
Diff_IL = 0.009;
% Differential shaft to right wheel intertial, kg-m2
Diff_IR = 0.009;
% Differential efficiency when driving, - 
Diff_ed = 0.99;
% Differential efficiency when coasting, - 
Diff_ec = 0.99;

% Driveline natural frequency, Hz
Driveline_wn = 9;
% Driveline damping ratio, -
Driveline_d = 0.9;
% Tire inertial, kg-m2
Iw = 0.8;


% Persistent transmission states
persistent gear;
persistent gear_state;
persistent gear_trigger;
if isempty(gear)
    gear = gr_init;
    gear_state = 0;
    gear_trigger = t;
end

% Current powertrain states
we = X(1);
Agrout = X(2);
wgrout = X(3);
wg = wg0*Diff_N;
Ag = Ag0*Diff_N;

% Shifting logic
if(t-gear_trigger < Trans1_legacy)
elseif(gear_state == 0)
    if(gear <= length(Trans1_u) && shiftState(Trans1_u{gear}, thr, wgrout/2/pi*60))
        gear_state = 1;
        gear_trigger = t;
    elseif(gear >= 2 && ~shiftState(Trans1_d{gear - 1}, thr, wgrout/2/pi*60))
        gear_state = -1;
        gear_trigger = t;
    end
elseif(gear_state == 1)
    if(shiftState(Trans1_u{gear}, thr, wgrout/2/pi*60))
        gear = gear + gear_state;
        gear_state = 0;
        gear_trigger = t;
    else
        gear_state = 0;
    end
elseif(gear_state == -1)
    if(~shiftState(Trans1_d{gear - 1}, thr, wgrout/2/pi*60))
        gear = gear + gear_state;
        gear_state = 0;
        gear_trigger = t;
    else
        gear_state = 0;
    end    
end

% transmission gear and input speed
Ntrans = Trans1_N(gear);
%Atco = Agrout * Ntrans;
wtco = wgrout * Ntrans;
% speed ratio
Stc = wtco / (abs(we)+1e-6); 
% engine torque
Te = intMap2(Eng1_thr, Eng1_rpm, Eng1, thr, we/2/pi*60); %(note: rad/s to rpm)
% torque converter torque
tki = intMap1(TC1_tki, Stc);
tr = intMap1(TC1_tr, Stc);
Ttcin = sign(tki)*(tki*we/2/pi*60).^2; 
Ttcout = tr * Ttcin;
% transmission efficiency and gear torque
if Ttcout >= 0
    Etrans = Trans1_ed(gear);
    Tgrout = Ttcout * Ntrans * Etrans;
else
    Etrans = Trans1_ec(gear);
    Tgrout = Ttcout * Ntrans / Etrans;
end
% Driveline inertials
I_trans = Trans1_I(gear); 
I_axle = Diff_Ishaft + (2*Iw + Diff_IL + Diff_IR)/Diff_N^2;
I_driveline_front_end = TC1_Ios*Ntrans^2 + 0.5*I_trans;
I_driveline_rear_end = 0.5*I_trans + I_axle;
I_driveline = 1.0/(1.0/I_driveline_front_end + 1.0/I_driveline_rear_end);
% Driveline stiffness
K_driveline = I_driveline * Driveline_wn^2;
% Driveline damping
D_driveline = I_driveline * 2*Driveline_wn*Driveline_d;
% Transmission output torque
Tg = K_driveline*(Agrout-Ag) + D_driveline*(wgrout-wg);
% Torque onto shaft with open differential
T_drv = zeros(2,1);
if Ttcout >= 0
    Ediff = Diff_ed;
    T_drv(1) = 0.5*Diff_N*Tg*Ediff;
    T_drv(2) = 0.5*Diff_N*Tg*Ediff;
else
    Ediff = Diff_ec;
    T_drv(1) = 0.5*Diff_N*Tg/Ediff;
    T_drv(2) = 0.5*Diff_N*Tg/Ediff;
end
% Powertrain dynamics
we_dot = (Te - Ttcin)/(Eng1_I + TC1_Iis);
Agrout_dot = wgrout;
wgrout_dot = (Tgrout - Tg)/I_driveline_front_end;
X_dot = zeros(3,1);
X_dot(1) = we_dot;
X_dot(2) = Agrout_dot;
X_dot(3) = wgrout_dot;
% Information
I_drv = (0.5*I_trans + Diff_Ishaft)*Diff_N^2/4;
gr = gear;
weng = we/2/pi*60;
wtran = wgrout/2/pi*60;
end

% Shift threshold judgement
function abv = shiftState(V, thr, rpm)
thr = min(max(thr, 0), 1);
rpm = min(max(rpm, 0), 9000);
for i = 1:size(V,1)-1
    if V(i+1,1) > thr; break; end
end
if rpm > V(i,2)*(V(i+1,1)-thr)/(V(i+1,1)-V(i,1))+V(i+1,2)*(thr-V(i,1))/(V(i+1,1)-V(i,1))
    abv = 1;
else
    abv = 0;
end
end

% 1D-Map interp
function v1 = intMap1(V, x0)
if x0 <= V(1,1)
    v1 = V(1,2);
elseif x0 >= V(end,1)
    v1 = V(end,2);
else
    for i = 1:size(V,1)-1
        if V(i+1,1) > x0; break; end
    end
    v1 = V(i,2)*(V(i+1,1)-x0)/(V(i+1,1)-V(i,1))+V(i+1,2)*(x0-V(i,1))/(V(i+1,1)-V(i,1));
end
end

% 2D-Map interp
function v2 = intMap2(x, y, V, x0, y0)
i2 = 0;
for i = 0:length(x)-1
    if x(i+1) > x0; i2 = 1; break; end
end
j2 = 0;
for j = 0:length(y)-1
    if y(j+1) > y0; j2 = 1; break; end
end
if i2 ~= 0 && i ~= 0
    if j2 ~= 0 && j~= 0
        v2 = (y(j+1)-y0)/(y(j+1)-y(j))*((x(i+1)-x0)/(x(i+1)-x(i))*V(j,i)+(x0-x(i))/(x(i+1)-x(i))*V(j,i+1))+...
            (y0-y(j))/(y(j+1)-y(j))*((x(i+1)-x0)/(x(i+1)-x(i))*V(j+1,i)+(x0-x(i))/(x(i+1)-x(i))*V(j+1,i+1));
    elseif j == 0
        v2 = (x(i+1)-x0)/(x(i+1)-x(i))*V(1,i)+(x0-x(i))/(x(i+1)-x(i))*V(1,i+1);
    else
        v2 = (x(i+1)-x0)/(x(i+1)-x(i))*V(j,i)+(x0-x(i))/(x(i+1)-x(i))*V(j,i+1);
    end
elseif i == 0
    if j2 ~= 0 && j~= 0
        v2 = (y(j+1)-y0)/(y(j+1)-y(j))*V(j,1)+(y0-y(j))/(y(j+1)-y(j))*V(j+1,1);
    elseif j == 0
        v2 = V(1,1);
    else
        v2 = V(j,1);
    end
else
    if j2 ~= 0 && j~= 0
        v2 = (y(j+1)-y0)/(y(j+1)-y(j))*V(j,i)+(y0-y(j))/(y(j+1)-y(j))*V(j+1,i);
    elseif j == 0
        v2 = V(1,i);
    else
        v2 = V(j,i);
    end
end
end

== matlab function VehRT_211219/Lane Keeping Basic/Lane Keeping Assistance/SMC_LKA_controler/MATLAB Function ==
  data: s input; y output
function y = fcn(s)
y=-0.7*s./(abs(s)+1)-(1-exp(-s))./(1+exp(-s))*0.4;
end

== matlab function VehRT_211219/Lane Keeping Basic/Lane Keeping Assistance/signal processing/prepoint_y/MATLAB Function1 ==
  data: local_x input; local_y input; xp output; local_yaw input; road_id input; yp output; preview_dis input
function [xp,yp] = fcn(local_x,local_y,local_yaw,road_id,preview_dis)
%#codegen
id1a = [149, 129, 122, 121, 118, 6];
id1b = [207, 193, 190, 196, 202, 188];
id1c = [276, 251, 254, 246, 281, 257];
id2a = [79, 441, 563, 564, 723];
id2b = [14, 24, 30, 27, 19];
id2c = [34, 46, 52, 49, 43];
if ismember(road_id, id1a)
     road1ax1 = 195.07312774;
     road1ay1 = -12.4755406379;
     road1ax2 =  207.1643981;
     road1ay2 = -13.2040925;
     cos_theta = (road1ax2-road1ax1)/sqrt((road1ax2-road1ax1).^2+(road1ay2-road1ay1).^2);
     sin_theta = (road1ay2-road1ay1)/sqrt((road1ax2-road1ax1).^2+(road1ay2-road1ay1).^2);
     theta = sign(sin_theta)*acos(cos_theta);
     segs1a=[cos_theta sin_theta;-sin_theta cos_theta]*[local_x-road1ax1; local_y-road1ay1];
     trans_x = segs1a(1);
     trans_y = segs1a(2);
     trans_yaw = local_yaw - theta;     
elseif ismember(road_id, id1b)
     road1ax1 = 165.5691223+0.004074493956;
     road1ay1 = -514.45065307+0.004437;
     road1ax2 = 163.015213012;
     road1ay2 = -519.8441772;
     cos_theta = (road1ax2-road1ax1)/sqrt((road1ax2-road1ax1).^2+(road1ay2-road1ay1).^2);
     sin_theta = (road1ay2-road1ay1)/sqrt((road1ax2-road1ax1).^2+(road1ay2-road1ay1).^2);
     theta = sign(sin_theta)*acos(cos_theta);
     segs1a=[cos_theta sin_theta;-sin_theta cos_theta]*[local_x-road1ax1; local_y-road1ay1];
     trans_x = segs1a(1);
     trans_y = segs1a(2);
     trans_yaw = local_yaw - theta;     
elseif ismember(road_id, id1c)     
     road1ax1 = -310.8804016+0.004074493956;
     road1ay1 = -279.1700134-0.004437;
     road1ax2 = -314.1051025;
     road1ay2 = -275.6842346;
     cos_theta = (road1ax2-road1ax1)/sqrt((road1ax2-road1ax1).^2+(road1ay2-road1ay1).^2);
     sin_theta = (road1ay2-road1ay1)/sqrt((road1ax2-road1ax1).^2+(road1ay2-road1ay1).^2);
     theta = sign(sin_theta)*acos(cos_theta);
     segs1a=[cos_theta sin_theta;-sin_theta cos_theta]*[local_x-road1ax1; local_y-road1ay1];
     trans_x = segs1a(1);
     trans_y = segs1a(2);
     trans_yaw = local_yaw - theta;    
elseif ismember(road_id, id2a)
     road1ax1 = 990.201171875;
     road1ay1 = -11.0457382;
     road1ax2 = 998.20233154;
     road1ay2 = -11.566880226;
     cos_theta = (road1ax2-road1ax1)/sqrt((road1ax2-road1ax1).^2+(road1ay2-road1ay1).^2);
     sin_theta = (road1ay2-road1ay1)/sqrt((road1ax2-road1ax1).^2+(road1ay2-road1ay1).^2);
     theta = sign(sin_theta)*acos(cos_theta);
     segs1a=[cos_theta sin_theta;-sin_theta cos_theta]*[local_x-road1ax1; local_y-road1ay1];
     trans_x = segs1a(1);
     trans_y = segs1a(2);
     trans_yaw = local_yaw - theta;    
elseif ismember(road_id, id2b)
     road1ax1 = 1018.778991699;
     road1ay1 = -535.160552979;
     road1ax2 = 1016.15411377;
     road1ay2 = -542.933654785;
     cos_theta = (road1ax2-road1ax1)/sqrt((road1ax2-road1ax1).^2+(road1ay2-road1ay1).^2);
     sin_theta = (road1ay2-road1ay1)/sqrt((road1ax2-road1ax1).^2+(road1ay2-road1ay1).^2);
     theta = sign(sin_theta)*acos(cos_theta);
     segs1a=[cos_theta sin_theta;-sin_theta cos_theta]*[local_x-road1ax1; local_y-road1ay1];
     trans_x = segs1a(1);
     trans_y = segs1a(2);
     trans_yaw = local_yaw - theta;    
elseif ismember(road_id, id2c)
     road1ax1 = 499.58631897;
     road1ay1 = -176.2607498;
     road1ax2 = 498.15455627;
     road1ay2 = -169.0533142;
     cos_theta = (road1ax2-road1ax1)/sqrt((road1ax2-road1ax1).^2+(road1ay2-road1ay1).^2);
     sin_theta = (road1ay2-road1ay1)/sqrt((road1ax2-road1ax1).^2+(road1ay2-road1ay1).^2);
     theta = sign(sin_theta)*acos(cos_theta);
     segs1a=[cos_theta sin_theta;-sin_theta cos_theta]*[local_x-road1ax1; local_y-road1ay1];
     trans_x = segs1a(1);
     trans_y = segs1a(2);
     trans_yaw = local_yaw - theta;    
else
     trans_x = 0;
     trans_y = -200;
     trans_yaw = 0;
end
yp=trans_y+preview_dis*sin(trans_yaw);
xp=trans_x+preview_dis*cos(trans_yaw);
end

== matlab function VehRT_211219/CEC Vehicle Dynamics 2021/CEC Vehicle Model 2021/Steering system/Steering Kinematics ==
  settings: updateMethod=DISCRETE
  data: sta input; stw output; chw output; Fx_gain output; Fy_gain output; Fz_gain output; Mz_gain output
function [stw, chw, Fx_gain, Fy_gain, Fz_gain, Mz_gain] = st(sta)
% Effective roling radius, m
Rw = 0.325; 
% 主销距离, kingpin lateral offset, m
dist = 0.075;
% 主销偏置, kingpin x coord., m
xcord = 0;
% 主销内倾角, kingpin inclination, deg
ang_ki = 13.5;
% 主销后倾角， kingpin caster angle, deg
ang_ca = 3;

% angle calculation functions
fun_cross = @(x,y) [x(2)*y(3)-x(3)*y(2), x(3)*y(1)-x(1)*y(3), x(1)*y(2)-x(2)*y(1)];
fun_dot = @(x,y) x(1)*y(1)+x(2)*y(2)+x(3)*y(3);
fun_rot = @(x,u,theta) cos(theta)*x + (1-cos(theta))*fun_dot(x, u)*u + sin(theta)*fun_cross(u, x);
fun_acos_p = @(x,u) acos((x(1)*u(1)+x(2)*u(2))/sqrt(x(1)^2+x(2)^2)/sqrt(u(1)^2+u(2)^2));

% reference vectors
z1 = [0,0,1];
y1 = [0,1,0];
% x1 = [1,0,0];
fc1 = [0,0,-Rw];
ac1 = [xcord, -dist, 0]; 
ad1 = [-sin(ang_ca/180*pi), -sin(ang_ki/180*pi), 1];
ad1 = ad1/norm(ad1);

z2 = [0,0,1];
y2 = [0,1,0];
% x2 = [1,0,0];
fc2 = [0,0,-Rw];
ac2 = [xcord, dist, 0]; 
ad2 = [-sin(ang_ca/180*pi), sin(ang_ki/180*pi), 1];
ad2 = ad2/norm(ad2);

% Geometric relationship
sta1 = sta(1);
sta2 = sta(2);

% rzd1 = fun_rot(z1, ad1, sta1);
ryd1 = fun_rot(y1, ad1, sta1);
% rxd1 = fun_rot(x1, ad1, sta1);
rfc1 = fun_rot(fc1-ac1, ad1, sta1)+ac1;
rc1 = fun_rot(-ac1, ad1, sta1)+ac1;

% rzd2 = fun_rot(z2, ad2, sta2);
ryd2 = fun_rot(y2, ad2, sta2);
% rxd2 = fun_rot(x2, ad2, sta2);
rfc2 = fun_rot(fc2-ac2, ad2, sta2)+ac2;
rc2 = fun_rot(-ac2, ad2, sta2)+ac2;

chw1  = atan(-ryd1(3)/sqrt(ryd1(1)^2+ryd1(2)^2));
chw2  = atan(-ryd2(3)/sqrt(ryd2(1)^2+ryd2(2)^2));

stw10 = fun_cross(-ac1,rc1-ac1)/norm(ac1)/norm(rc1-ac1);
stw1 = asin(stw10(3));
stw20 = fun_cross(-ac2,rc2-ac2)/norm(ac2)/norm(rc2-ac2);
stw2 = asin(stw20(3));

zd1 = z1;
yd1 = [-sin(stw1), cos(stw1), 0];
xd1 = [cos(stw1), sin(stw1), 0];
zd2 = z2;
yd2 = [-sin(stw2), cos(stw2), 0];
xd2 = [cos(stw2), sin(stw2), 0];


% Kinematic relationship
Fx_gain1 = ad1*(fun_cross(rfc1-ac1, xd1))';
Fy_gain1 = ad1*(fun_cross(rfc1-ac1, yd1))';
Fz_gain1 = ad1*(fun_cross(rfc1-ac1, zd1))';
Mz_gain1 = ad1*zd1';
Fx_gain2 = ad2*(fun_cross(rfc2-ac2, xd2))';
Fy_gain2 = ad2*(fun_cross(rfc2-ac2, yd2))';
Fz_gain2 = ad2*(fun_cross(rfc2-ac2, zd2))';
Mz_gain2 = ad2*zd1';

% outputs
stw = [stw1, stw2];
chw = [chw1, chw2];
Fx_gain =[Fx_gain1, Fx_gain2];
Fy_gain =[Fy_gain1, Fy_gain2];
Fz_gain =[Fz_gain1, Fz_gain2];
Mz_gain =[Mz_gain1, Mz_gain2];
end
